simulink model "plant_block"  (R2013a)
settings: Solver=ode1  StartTime=0.0  StopTime=60  RelTol=1e-3
libraries: simulink x1
settings Model: SimulationMode=external  ExtModeTrigDuration=50000  Creator=Dro  LastModifiedBy=s4358762
settings DataIOCC: LimitDataPoints=off  SignalLoggingSaveFormat=ModelDataLogs  SignalLoggingName=sigsOut
settings OptimizationCC: ExpressionDepthLimit=2147483647  InitFltsAndDblsToZero=on
settings DebuggingCC: SaveWithParameterizedLinksMsg=none  SignalResolutionControl=TryResolveAllWithWarning  SolverPrmCheckMsg=none  MultiTaskDSMMsg=warning  MultiTaskCondExecSysMsg=none  FcnCallInpInsideContextMsg=UseLocalSettings  StrictBusMsg=None
settings RTWCC: SystemTargetFile=rtwin.tlc  TemplateMakefile=rtwin.tmf  Description=Real-Time Windows Target  ProcessScript=rtwin_make_rtw_hook  IncludeERTFirstTime=on
settings RTWinTargetCC: TargetFcnLib=ansi_tfl_tmw.mat  TargetLibSuffix=_rtwin.lib  TargetPreCompLibLocation=C:\Program Files\MATLAB\R2013a\toolbox\rtw\targets\rtwin\lib\win64  CodeReplacementLibrary=ANSI_C  ModelReferenceCompliant=off  CompOptLevelCompliant=off  RTWinDir=C:/PROGRA~1/MATLAB/R2013a/toolbox/rtw/targets/rtwin  TargetArch=win64

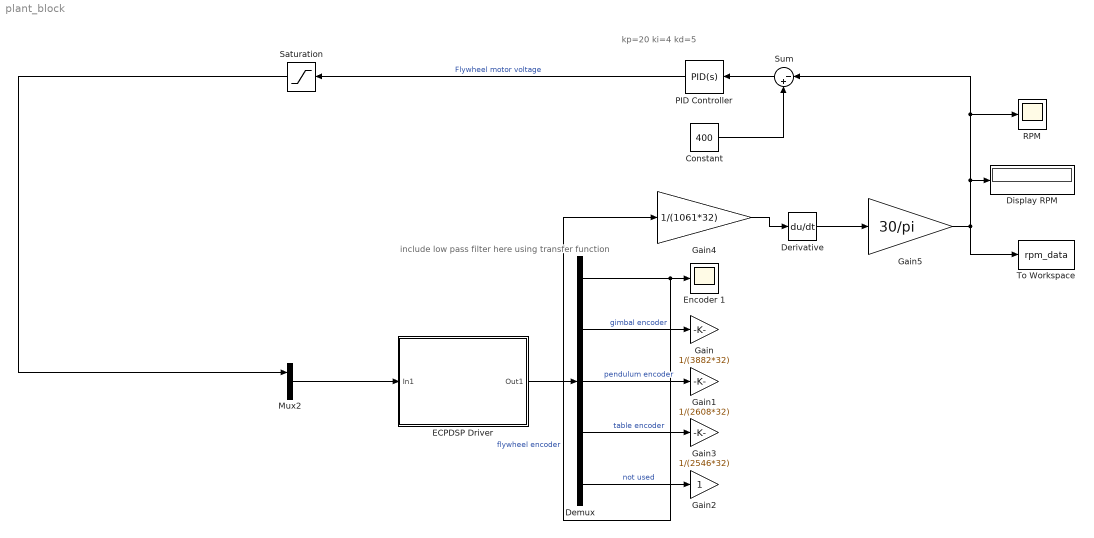
== system plant_block ==
  note: include low pass filter here
      | using transfer function
  note: kp=20
      | ki=4
      | kd=5
  Constant : Constant  Value=400
  Demux : Demux  Outputs=5
  Derivative : Derivative
  Display RPM : Display
  ECPDSP Driver : Subsystem  mask{BaseAddr='0xC000', STime=0.008, TimeOutPer=500, HWAccess=on}
      mask prompts: BaseAddr "Base I/O Address"; STime "Sample Time (Sec)"; TimeOutPer "Timeout Period (500 ~ 2000)"; HWAccess "Hardware Access"
      mask Display: color('black');disp('ECPDSP Driver\n upto\n 4 Encs(ADC Channels)\n and 2 Dacs')
  Encoder 1 : Scope
      settings: YMin=1.5e+06  YMax=8.5e+06  SaveName=ScopeData3
  Gain : Gain  Gain=1/(3882*32)
  Gain1 : Gain  Gain=1/(2608*32)
  Gain2 : Gain
  Gain3 : Gain  Gain=1/(2546*32)
  Gain4 : Gain  Gain=1/(1061*32)
  Gain5 : Gain  Gain=30/pi
  Mux2 : Mux  Inputs=2
  PID Controller : simulink/Continuous/PID Controller  Controller=PID  TimeDomain=Continuous-time  SampleTime=1  IntegratorMethod=Forward Euler  FilterMethod=Forward Euler  Form=Parallel  P=20  I=4  D=5  N=100  InitialConditionSource=internal  InitialConditionForIntegrator=0  InitialConditionForFilter=0  ExternalReset=none  LimitOutput=off  UpperSaturationLimit=inf  LowerSaturationLimit=-inf  LinearizeAsGain=on  AntiWindupMode=none  Kb=1  TrackingMode=off  Kt=1  PParamMin=[]  PParamMax=[]  IParamMin=[]  IParamMax=[]  DParamMin=[]  DParamMax=[]  NParamMin=[]  NParamMax=[]  KbParamMin=[]  KbParamMax=[]  KtParamMin=[]  KtParamMax=[]  POutMin=[]  POutMax=[]  IOutMin=[]  IOutMax=[]  DOutMin=[]  DOutMax=[]  NOutMin=[]  NOutMax=[]  KbOutMin=[]  KbOutMax=[]  KtOutMin=[]  KtOutMax=[]  IntegratorOutMin=[]  IntegratorOutMax=[]  FilterOutMin=[]  FilterOutMax=[]  SumOutMin=[]  SumOutMax=[]  SumI1OutMin=[]  SumI1OutMax=[]  SumI2OutMin=[]  SumI2OutMax=[]  SumI3OutMin=[]  SumI3OutMax=[]  SumDOutMin=[]  SumDOutMax=[]  SaturationOutMin=[]  SaturationOutMax=[]  IntegratorContinuousStateAttributes=''  IntegratorStateMustResolveToSignalObject=off  IntegratorRTWStateStorageClass=Auto  FilterContinuousStateAttributes=''  FilterStateMustResolveToSignalObject=off  FilterRTWStateStorageClass=Auto
  RPM : Scope
      settings: YMin=125  YMax=375
  Saturation : Saturate  UpperLimit=32000  LowerLimit=-32000
  Sum : Sum  Inputs=|-+
  To Workspace : ToWorkspace  VariableName=rpm_data  SampleTime=-1  SaveFormat=Timeseries
  wires:
  ECPDSP Driver/1(Out1) -> Demux/1
  Demux/1 -> Gain4/1, Encoder 1/1  "flywheel encoder"
  Mux2/1 -> ECPDSP Driver/1(In1)
  PID Controller/1 -> Saturation/1  "Flywheel motor voltage"
  ? -> Mux2/2  "gimbal motor voltage"
  Demux/2 -> Gain/1  "gimbal encoder"
  Demux/3 -> Gain1/1  "pendulum encoder"
  Demux/4 -> Gain3/1  "table encoder"
  Demux/5 -> Gain2/1  "not used"
  Gain4/1 -> Derivative/1
  Derivative/1 -> Gain5/1
  Gain5/1 -> To Workspace/1, Display RPM/1, RPM/1, Sum/1
  Constant/1 -> Sum/2
  Sum/1 -> PID Controller/1
  Saturation/1 -> Mux2/1

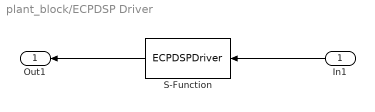
== system plant_block/ECPDSP Driver ==
  In1 : Inport
  S-Function : S-Function  FunctionName=ECPDSPDriver  Parameters=BaseAddr,STime,TimeOutPer,HWAccess  EnableBusSupport=off
  Out1 : Outport
  wires:
  In1/1 -> S-Function/1
  S-Function/1 -> Out1/1
